simulink model "Tugas1FLCMotor"  (R2021a)
settings: Solver=VariableStepAuto  StartTime=0.0  StopTime=5  RelTol=1e-3
undefined symbols (not defined in the file): DiscIntNeverNeededParam
libraries: spsCurrentMeasurementLib x3, spsUniversalBridgeLib x2, spsACVoltageSourceLib x1, spsAsynchronousMachinepuUnitsLib x1, spsSeriesRLCBranchLib x1, powerlib_extras x1, fuzblock x1, spsVoltageMeasurementLib x1, spspowerguiLib x1
settings Model: Creator=Azriel  LastModifiedBy=Azriel

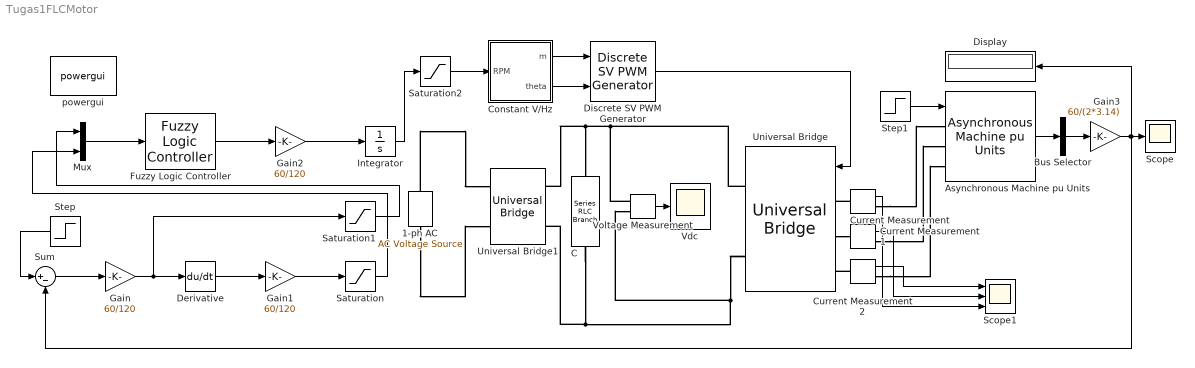
== system Tugas1FLCMotor ==
  1-ph AC : spsACVoltageSourceLib/AC Voltage Source  Amplitude=464.6702  Phase=0  Frequency=50  SampleTime=0  Measurements=None  BusType=swing  Pref=10e3  Qref=0  Qmin=-inf  Qmax=+inf
  Asynchronous Machine pu Units : spsAsynchronousMachinepuUnitsLib/Asynchronous Machine pu Units  RotorType=Squirrel-cage  PresetModel=No  MechanicalLoad=Torque Tm  ShowDetailedParameters=on  ReferenceFrame=Synchronous  Units=pu  MeasurementBus=off  NominalParameters=[3730 460 60]  VoltageRatio=1  Stator=[0.01965 0.0397]  Rotor=[0.01909 0.0397]  Cage1=[0.01909 0.0397]  Cage2=[0.01909 0.0397]  Lm=1.354  Mechanical=[0.09526 0.05479 2]  PolePairs=2  InitialConditions="[ 1,0   0,0,0   0,0,0 ]"  SimulateSaturation=off  Saturation="[0.212,0.4201,0.8125,1.0979,1.4799,2.2457,3.2586,4.5763,6.4763 ;   0.5,0.7,0.9,1,1.1,1.2 ,1.3,1.4,1.5]"  LoadFlowParameters=0  TsPowergui=0  TsBlock=-1  IterativeModel=Trapezoidal non iterative  IterativeDiscreteModel=Trapezoidal non iterative  Pmec=0
      settings: SourceProductBaseCode=PS
  Bus Selector : BusSelector  OutputSignals=Mechanical.Rotor speed (wm)  OutputAsBus=on
  C : spsSeriesRLCBranchLib/Series RLC Branch  LConnTagsString=__new0  RConnTagsString=__new0  BranchType=C  Resistance=1  Inductance=1e-3  SetiL0=off  InitialCurrent=0  Capacitance=47e-3  Setx0=off  InitialVoltage=0  Measurements=None
  Constant V/Hz : Subsystem
  Current Measurement : spsCurrentMeasurementLib/Current Measurement  PhasorSimulation=off  OutputType=Complex  PSBequivalent=0
  Current Measurement1 : spsCurrentMeasurementLib/Current Measurement  PhasorSimulation=off  OutputType=Complex  PSBequivalent=0
  Current Measurement2 : spsCurrentMeasurementLib/Current Measurement  PhasorSimulation=off  OutputType=Complex  PSBequivalent=0
  Derivative : Derivative
  Discrete SV PWM Generator : powerlib_extras/Discrete  Control Blocks/Discrete SV PWM Generator  InputType=Magnitude-Angle (rad)  SwitchingPattern=Pattern #1  Fc=1980  ParUref=[0.8 -30 50]  Ts=0.5
      settings: SourceProductBaseCode=PS
  Display : Display
  Fuzzy Logic Controller : fuzblock/Fuzzy Logic  Controller  FIS='trop_3.fis'  OutputSampleNumber=101  DataType=double  FuzzifiedInputs=off  RuleFiringStrengths=off  RuleOutputs=off  AggregatedOutputs=off  SimulateUsing=Interpreted execution  OutOfRangeInputValueMessage=warning  NoRuleFiredMessage=warning  EmptyOutputFuzzySetMessage=warning
  Gain : Gain  Gain=60/120
  Gain1 : Gain  Gain=60/120
  Gain2 : Gain  Gain=60/120
  Gain3 : Gain  Gain=60/(2*3.14)
  Integrator : Integrator
  Mux : Mux  Inputs=2
  Saturation : Saturate
  Saturation1 : Saturate
  Saturation2 : Saturate
  Scope : Scope
  Scope1 : Scope  NumInputPorts=3
  Step : Step  Time=0  Before=2000  After=0  SampleTime=5
  Step1 : Step  Time=0  Before=2500  After=0  SampleTime=5
  Sum : Sum  Inputs=|+-
  Universal Bridge : spsUniversalBridgeLib/Universal Bridge  Arms=3  SnubberResistance=1e5  SnubberCapacitance=inf  Device=MOSFET / Diodes  Ron=1e-3  Lon=0  ForwardVoltages="[  0  0  ]"  ForwardVoltage=0  GTOparameters=[ 10e-6 , 20e-6 ]  IGBTparameters=[ 1e-6 , 2e-6 ]  Measurements=None  Measurements_2=None  converterType=Rectifier
  Universal Bridge1 : spsUniversalBridgeLib/Universal Bridge  Arms=2  SnubberResistance=1e5  SnubberCapacitance=inf  Device=Diodes  Ron=1e-3  Lon=0  ForwardVoltages="[  0  0  ]"  ForwardVoltage=0  GTOparameters=[ 10e-6 , 20e-6 ]  IGBTparameters=[ 1e-6 , 2e-6 ]  Measurements=None  Measurements_2=None  converterType=Rectifier
  Vdc : Scope
  Voltage Measurement : spsVoltageMeasurementLib/Voltage Measurement  PhasorSimulation=off  OutputType=Complex  PSBequivalent=0
  powergui : spspowerguiLib/powergui  Priority=1  SimulationMode=Continuous  SampleTime=0.5  frequency=60  Iterations=50  frequencyindice=50  Pbase=100e6  ErrMax=1e-4  UnitsV=kV  UnitsW=MW  buscounter=0  FunctionMessages=off  echomessages=off  EnableUseOfTLC=off  CurrentSourceSwitches=off  DisableSnubberDevices=off  DisableRonSwitches=off  DisableVfSwitches=off  DisplayEquations=off  AutomaticDiscreteSolvers=off  SolverType=Tustin/Backward Euler (TBE)  Interpol=off  ExternalGateDelay=off  methode=off  Ts=0  x0status=blocks  SPID=off  SwTol=0  HookPort=off  NonlinearTolerance=1e-4  nMaxIteration=100  ContinueOnMaxIteration=off  RestoreLinks=warning  ResistiveCurrentMeasurement=off  Frange=[0:2:500]  Ylog=off  Xlog=on  ShowGrid=off  save=off  variable=ZData  structure=vl  ZoomFFT=off  StartTime=1  cycles=10  DisplayStyle=1  fundamental=61  FreqAxis=off  MaxFrequency=1000  frequencyindicesteady=1  RmsSteady=1  display=off
  wires:
  Step/1 -> Sum/1
  Sum/1 -> Gain/1
  Gain/1 -> Saturation1/1, Derivative/1
  Derivative/1 -> Gain1/1
  Gain1/1 -> Saturation/1
  Saturation1/1 -> Mux/1
  Saturation/1 -> Mux/2
  Mux/1 -> Fuzzy Logic Controller/1
  Fuzzy Logic Controller/1 -> Gain2/1
  Gain2/1 -> Integrator/1
  Integrator/1 -> Saturation2/1
  Gain3/1 -> Display/1, Sum/2, Scope/1
  Step1/1 -> Asynchronous Machine pu Units/1
  Constant V/Hz/1(m) -> Discrete SV PWM Generator/1
  Constant V/Hz/2(theta) -> Discrete SV PWM Generator/2
  Saturation2/1 -> Constant V/Hz/1(RPM)
  Voltage Measurement/1 -> Vdc/1
  Discrete SV PWM Generator/1 -> Universal Bridge/1
  Asynchronous Machine pu Units/1 -> Bus Selector/1
  Bus Selector/1 -> Gain3/1
  Current Measurement2/1 -> Scope1/1
  Current Measurement1/1 -> Scope1/2
  Current Measurement/1 -> Scope1/3
  connections:
  Universal Bridge/RConn2 -- Universal Bridge1/RConn2 -- C/RConn1 -- Voltage Measurement/LConn2
  Voltage Measurement/LConn1 -- Universal Bridge/RConn1 -- Universal Bridge1/RConn1 -- C/LConn1
  1-ph AC/LConn1 -- Universal Bridge1/LConn2
  1-ph AC/RConn1 -- Universal Bridge1/LConn1
  Current Measurement/LConn1 -- Universal Bridge/LConn1
  Universal Bridge/LConn2 -- Current Measurement1/LConn1
  Current Measurement2/LConn1 -- Universal Bridge/LConn3
  Current Measurement/RConn1 -- Asynchronous Machine pu Units/LConn1
  Current Measurement1/RConn1 -- Asynchronous Machine pu Units/LConn2
  Current Measurement2/RConn1 -- Asynchronous Machine pu Units/LConn3

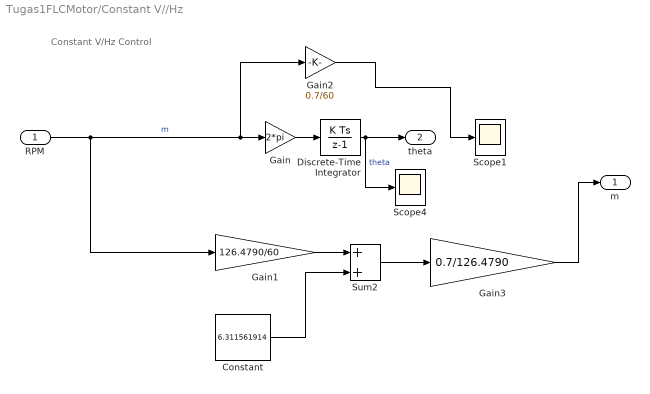
== system Tugas1FLCMotor/Constant V//Hz ==
  note: Constant V/Hz
      | Control
  RPM : Inport
  Constant : Constant  Value=6.311561914
  Discrete-Time Integrator : DiscreteIntegrator  ICPrevOutput=DiscIntNeverNeededParam  ICPrevScaledInput=DiscIntNeverNeededParam
  Gain : Gain  Gain=2*pi  SaturateOnIntegerOverflow=on  OutDataTypeStr=Inherit: Same as input  ParamDataTypeStr=Inherit: Same as input
  Gain1 : Gain  Gain=126.4790/60
  Gain2 : Gain  Gain=0.7/60  SaturateOnIntegerOverflow=on  OutDataTypeStr=Inherit: Same as input  ParamDataTypeStr=Inherit: Same as input
  Gain3 : Gain  Gain=0.7/126.4790
  Scope1 : Scope
  Scope4 : Scope
  Sum2 : Sum
  m : Outport
  theta : Outport  Port=2
  wires:
  Gain/1 -> Discrete-Time Integrator/1
  RPM/1 -> Gain/1, Gain2/1, Gain1/1  "m"
  Discrete-Time Integrator/1 -> theta/1, Scope4/1  "theta"
  Gain2/1 -> Scope1/1
  Gain1/1 -> Sum2/1
  Constant/1 -> Sum2/2
  Sum2/1 -> Gain3/1
  Gain3/1 -> m/1
